simulink model "model"  (R2023a)
settings: Solver=VariableStepAuto  StartTime=0.0  StopTime=10.0  RelTol=1e-3
libraries: simulink x1
settings Model: Creator=artemii  LastModifiedBy=Theomur

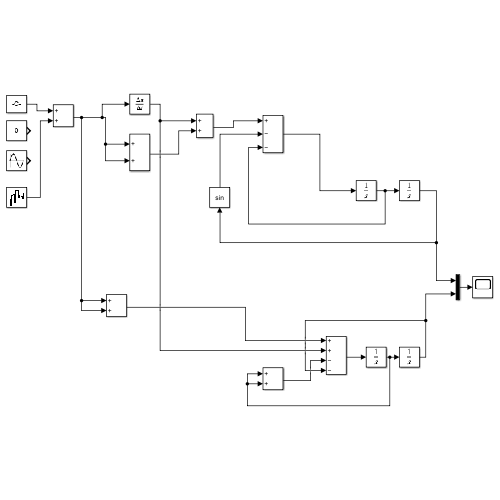
[thumbnail: Simulink's stored preview of the top-level diagram]
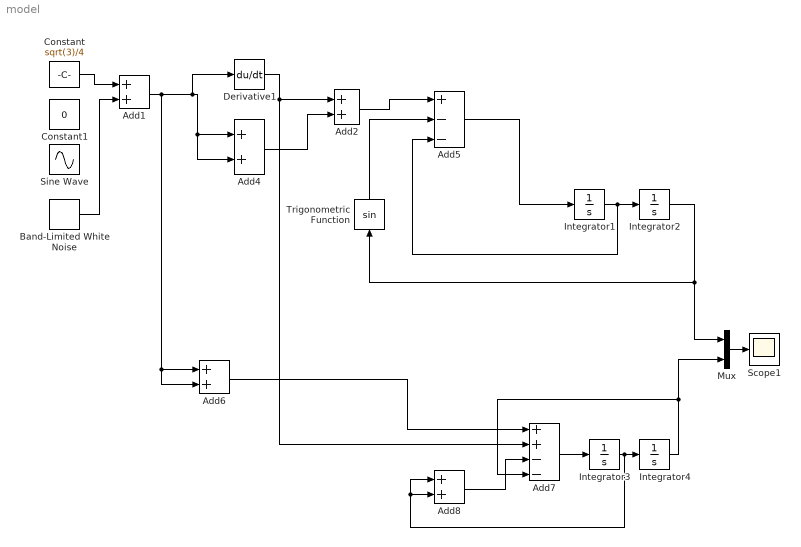
== system model ==
  Add{1..2,4,6,8} (5 alike) : Sum
  Add5 : Sum  Inputs=+--
  Add7 : Sum  Inputs=++--
  Band-Limited White Noise : simulink/Sources/Band-Limited White Noise  Cov=[0.1]  Ts=0.1  seed=[12345]
  Constant : Constant  Value=sqrt(3)/4
  Constant1 : Constant  Value=0
  Derivative1 : Derivative
  Integrator{1..4} (4 alike) : Integrator
  Mux : Mux  Inputs=2
  Scope1 : Scope
  Sine Wave : Sin  SampleTime=0
  Trigonometric Function : Trigonometry
  wires:
  Constant/1 -> Add1/1
  Mux/1 -> Scope1/1
  Band-Limited White Noise/1 -> Add1/2
  Add1/1 -> Add6/2, Add6/1, Derivative1/1, Add4/2, Add4/1
  Derivative1/1 -> Add7/2, Add2/1
  Add4/1 -> Add2/2
  Add2/1 -> Add5/1
  Integrator1/1 -> Add5/3, Integrator2/1
  Add5/1 -> Integrator1/1
  Integrator2/1 -> Mux/1, Trigonometric Function/1
  Trigonometric Function/1 -> Add5/2
  Add7/1 -> Integrator3/1
  Add6/1 -> Add7/1
  Add8/1 -> Add7/3
  Integrator3/1 -> Add8/1, Add8/2, Integrator4/1
  Integrator4/1 -> Mux/2, Add7/4
